simulink model "CIMA_FBL"  (R2023b)
settings: Solver=VariableStepAuto  StartTime=0.0  StopTime=30  RelTol=1e-6
values from neighbouring files (symbols this model uses):
  a = 10    [CIMA_Classification_Stab_Equilibrium.m]    (also in CIMA_Control_routine.m)
  b = b_vec(i)    [CIMA_Classification_Stab_Equilibrium.m]    (also in CIMA_Control_routine.m = 2)
  x0 = [x1_eq+0.5; x2_eq+0.2]    [CIMA_Control_routine.m]
settings Model: Creator=user  LastModifiedBy=user

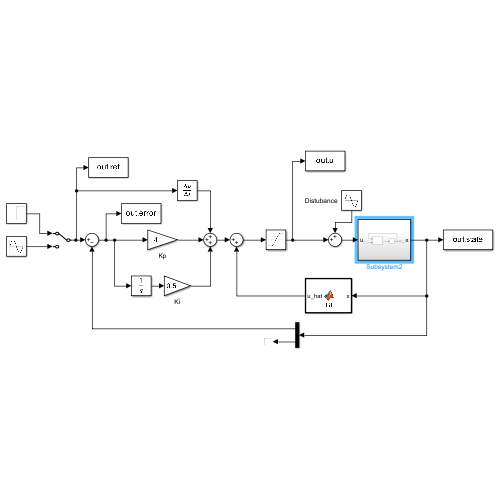
[thumbnail: Simulink's stored preview of the top-level diagram]
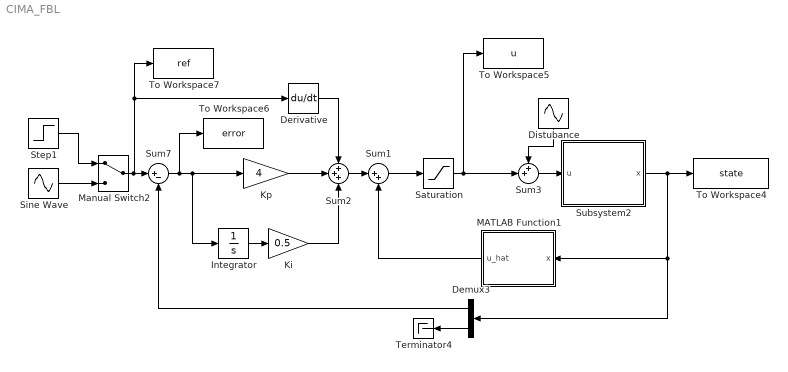
== system CIMA_FBL ==
  Demux3 : Demux  Outputs=2
  Derivative : Derivative
  Distubance : Sin  Amplitude=0.6*0  SampleTime=0
  Integrator : Integrator
  Ki : Gain  Gain=0.5
  Kp : Gain  Gain=4
  MATLAB Function1 : MATLAB Function  TreatAsAtomicUnit=on
  Manual Switch2 : ManualSwitch
  Saturation : Saturate  UpperLimit=20  LowerLimit=0
  Sine Wave : Sin  Amplitude=0.5  Bias=5  Frequency=2  SampleTime=0
  Step1 : Step  Time=0  After=5  SampleTime=0
  Subsystem2 : Subsystem
  Sum1 : Sum  Inputs=|++
  Sum2 : Sum  Inputs=+++
  Sum3 : Sum  Inputs=++|
  Sum7 : Sum  Inputs=|+-
  Terminator4 : Terminator
  To Workspace4 : ToWorkspace  VariableName=state  SaveFormat=Structure With Time  SampleTime=-1
  To Workspace5 : ToWorkspace  VariableName=u  SaveFormat=Structure With Time  SampleTime=-1
  To Workspace6 : ToWorkspace  VariableName=error  SaveFormat=Structure With Time  SampleTime=-1
  To Workspace7 : ToWorkspace  VariableName=ref  SaveFormat=Structure With Time  SampleTime=-1
  wires:
  Manual Switch2/1 -> To Workspace7/1, Derivative/1, Sum7/1
  Sum7/1 -> To Workspace6/1, Kp/1, Integrator/1
  Subsystem2/1(x) -> To Workspace4/1, Demux3/1, MATLAB Function1/1(x)
  Demux3/1 -> Sum7/2
  Demux3/2 -> Terminator4/1
  Kp/1 -> Sum2/2
  Derivative/1 -> Sum2/1
  Integrator/1 -> Ki/1
  Ki/1 -> Sum2/3
  Sum2/1 -> Sum1/1
  MATLAB Function1/1(u_hat) -> Sum1/2
  Sum1/1 -> Saturation/1
  Saturation/1 -> To Workspace5/1, Sum3/2
  Sum3/1 -> Subsystem2/1(u)
  Distubance/1 -> Sum3/1
  Step1/1 -> Manual Switch2/1
  Sine Wave/1 -> Manual Switch2/2

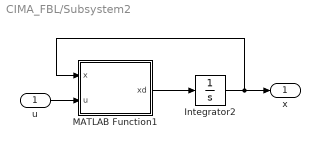
== system CIMA_FBL/Subsystem2 ==
  u : Inport
  Integrator2 : Integrator  InitialCondition=x0  UpperSaturationLimit=18
  MATLAB Function1 : MATLAB Function  TreatAsAtomicUnit=on
  x : Outport
  wires:
  MATLAB Function1/1(xd) -> Integrator2/1
  Integrator2/1 -> x/1, MATLAB Function1/1(x)
  u/1 -> MATLAB Function1/2(u)

== matlab function CIMA_FBL/MATLAB Function1 ==
  data: x input; u_hat output; a parameter
function u_hat = FBL(x, a)

u_hat = - (a - x(1) - 4*x(1)*x(2)/(1 + x(1)^2));

== matlab function CIMA_FBL/Subsystem2/MATLAB Function1 ==
  data: x input; u input; xd output; a parameter; b parameter
function xd = cima(x, u, a, b)

xd1 = a -x(1) - 4*x(1)*x(2)/(1 + x(1)^2) + u; 
xd2 = b*x(1)*(1 - x(2)/(1 + x(1)^2)); 

%Parameter uncertanties 10%
% xd1 = 0.9*a -x(1) - 4*x(1)*x(2)/(1 + x(1)^2) + u; 
% xd2 = 1.1*b*x(1)*(1 - x(2)/(1 + x(1)^2)); 

%Parameter uncertanties 20%
% xd1 = 1.2*a -x(1) - 4*x(1)*x(2)/(1 + x(1)^2) + u; 
% xd2 = 0.8*b*x(1)*(1 - x(2)/(1 + x(1)^2)); 

xd = [xd1;xd2];
